simulink library "CarLib"  (R2017b)
settings: Solver=VariableStepAuto  StartTime=0.0  StopTime=10.0  RelTol=1e-3
settings Model: Creator=Seb  LastModifiedBy=Seb

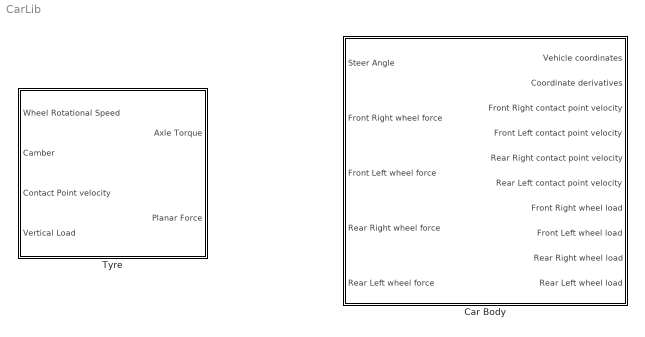
== system CarLib ==
  Car Body : Subsystem  mask{x0=[0;0;0; 0;0;0; 0;0;0; 0;0;0], paramsfile='myparams.mat'}
      mask prompts: x0 "Initial State"; paramsfile "Parameters File"
      mask init:
      | try
      | load(paramsfile);
      | catch
      |     warning(['Parameters file "', paramsfile, '" not found']);   
      |     return
      | end
  Tyre : Subsystem  mask{tirfilename='mytyre.tir'}
      mask prompts: tirfilename ".TIR file"
      mask init:
      | % Load TIR File
      | try
      | TIRparam = loadTIR(tirfilename);
      | catch
      |     warning(['File "', tirfilename, '" not found']);   
      |     return
      | end
      | % Keep only the numetic fields (avoir simulink errors) 
      | % and save it into PARAMETER_SOURCE
      | fn = fieldnames(TIRparam);
      | for k = 1:numel(fn)
      |    
      |     v = TIRparam.(fn{k});
      |     if(isnumeric(v))
      |         PAC96coeffs.(fn{k}) = v;
      |     end
      |    
      | end

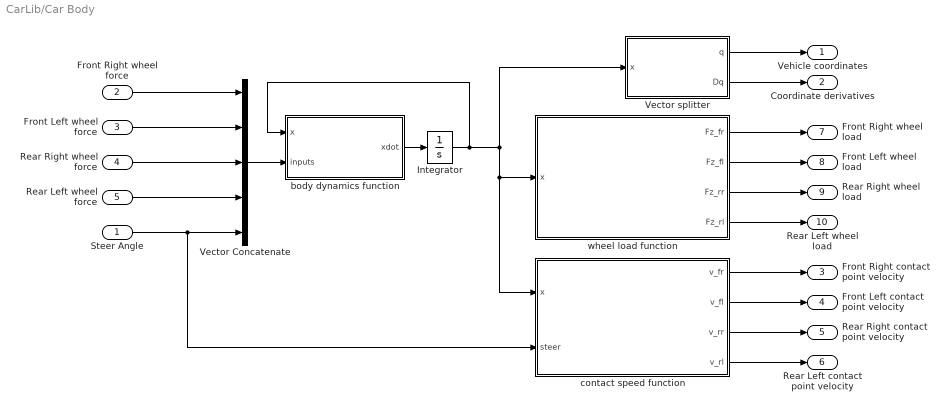
== system CarLib/Car Body ==
  Steer Angle : Inport
  Front Right wheel force : Inport  Port=2  PortDimensions=[2,1]
  Front Left wheel force : Inport  Port=3  PortDimensions=[2,1]
  Rear Right wheel force : Inport  Port=4  PortDimensions=[2,1]
  Rear Left wheel force : Inport  Port=5  PortDimensions=[2,1]
  Integrator : Integrator  InitialCondition=x0
  Vector Concatenate : Concatenate  NumInputs=5
  Vector splitter : MATLAB Function  TreatAsAtomicUnit=on
  body dynamics function : MATLAB Function  TreatAsAtomicUnit=on
  "contact speed function " : MATLAB Function  TreatAsAtomicUnit=on
  wheel load function : MATLAB Function  TreatAsAtomicUnit=on
  Vehicle coordinates : Outport
  "Coordinate derivatives " : Outport  Port=2
  Front Right contact point velocity : Outport  Port=3
  "Front Left contact point velocity " : Outport  Port=4
  "Rear Right contact point velocity " : Outport  Port=5
  Rear Left contact point velocity : Outport  Port=6
  Front Right wheel load : Outport  Port=7  PortDimensions=1
  Front Left wheel load : Outport  Port=8  PortDimensions=1
  Rear Right wheel load : Outport  Port=9  PortDimensions=1
  Rear Left wheel load : Outport  Port=10  PortDimensions=1
  wires:
  Front Right wheel force/1 -> Vector Concatenate/1
  Vector Concatenate/1 -> body dynamics function/2(inputs)
  body dynamics function/1(xdot) -> Integrator/1
  Integrator/1 -> Vector splitter/1(x), wheel load function/1(x), "contact speed function "/1(x), body dynamics function/1(x)
  "contact speed function "/1(v_fr) -> Front Right contact point velocity/1
  Front Left wheel force/1 -> Vector Concatenate/2
  Rear Right wheel force/1 -> Vector Concatenate/3
  Rear Left wheel force/1 -> Vector Concatenate/4
  Steer Angle/1 -> Vector Concatenate/5, "contact speed function "/2(steer)
  "contact speed function "/2(v_fl) -> "Front Left contact point velocity "/1
  "contact speed function "/3(v_rr) -> "Rear Right contact point velocity "/1
  "contact speed function "/4(v_rl) -> Rear Left contact point velocity/1
  wheel load function/1(Fz_fr) -> Front Right wheel load/1
  wheel load function/3(Fz_rr) -> Rear Right wheel load/1
  wheel load function/2(Fz_fl) -> Front Left wheel load/1
  wheel load function/4(Fz_rl) -> Rear Left wheel load/1
  Vector splitter/1(q) -> Vehicle coordinates/1
  Vector splitter/2(Dq) -> "Coordinate derivatives "/1

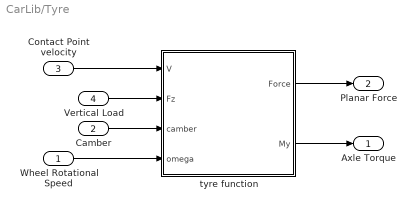
== system CarLib/Tyre ==
  Wheel Rotational Speed : Inport
  Camber : Inport  Port=2
  Contact Point velocity : Inport  Port=3
  Vertical Load : Inport  Port=4
  "tyre function " : MATLAB Function  TreatAsAtomicUnit=on
  Axle Torque : Outport
  Planar Force : Outport  Port=2
  wires:
  Wheel Rotational Speed/1 -> "tyre function "/4(omega)
  Vertical Load/1 -> "tyre function "/2(Fz)
  Contact Point velocity/1 -> "tyre function "/1(V)
  Camber/1 -> "tyre function "/3(camber)
  "tyre function "/1(Force) -> Planar Force/1
  "tyre function "/2(My) -> Axle Torque/1

== matlab function CarLib/Car Body/body dynamics function ==
  data: xdot output; x input; inputs input; parameters parameter
function xdot = dynamics(x, inputs, parameters)

xdot = C210BodyDynamicsFunction(x, inputs, parameters);

end

== matlab function CarLib/Tyre/tyre function  ==
  data: V input; Force output; Fz input; camber input; omega input; My output; PAC96coeffs parameter
function [Force, My] = tyre(V, Fz, camber, omega, PAC96coeffs)

RE = V(1,:)./omega;
R0 = PAC96coeffs.UNLOADED_RADIUS;

SL = R0./RE;
SA = atan(-V(2,:)./V(1,:));

[Fx, Fy, ~, ~] = C310pacejka96(SL, SA, camber, Fz, PAC96coeffs);

My = R0.*Fy;

Force = [Fx;Fy];

end

== matlab function CarLib/Car Body/contact speed function  ==
  data: v_fr output; v_fl output; v_rr output; v_rl output; x input; steer input; parameters parameter
function [v_fr, v_fl, v_rr, v_rl] = computeContactPointVelocities(x, steer, parameters)
    CPV  = C230ContactPointVelocitiesFunction(x,steer,parameters);
    v_fr = CPV(1:2,1);
    v_fl = CPV(1:2,2);
    v_rr = CPV(1:2,3);
    v_rl = CPV(1:2,4);
end

== matlab function CarLib/Car Body/wheel load function ==
  data: x input; Fz_fr output; Fz_fl output; Fz_rr output; Fz_rl output; parameters parameter
function [Fz_fr, Fz_fl, Fz_rr, Fz_rl] = computeWheelLoads(x,parameters)
    FZ = C220WheelLoadsFunction(x,parameters);
    Fz_fr = FZ(:,1);
    Fz_fl = FZ(:,2);
    Fz_rr = FZ(:,3);
    Fz_rl = FZ(:,4);
end

== matlab function CarLib/Car Body/Vector splitter ==
  data: x input; q output; Dq output
function [q,Dq] = split(x)
    q = x(1:6);
    Dq = x(7:12);
end
